simulink model "Modell_V5"  (R2014a)
settings: Solver=ode45  StartTime=0.0  StopTime=2  RelTol=1e-10
values from neighbouring files (symbols this model uses):
  AP = [pi 0 pi 0]'    [testscript.m]
  M_AP = 0    [testscript.m]
  stPendel = block.DialogPrm(1).Data    [systemPendel_V3.m]    (also in testscript.m = ladePendel())
  stTraj = berechneTrajektorie( stPendel, Q, R, T)    [testscript.m]
  x0 = block.DialogPrm(2).Data    [systemPendel_V3.m]    (also in testscript.m = [ 0 0 0 0]')
settings Model: Creator=asacakli  LastModifiedBy=Andreas
settings DataIOCC: SaveFormat=Dataset
settings OptimizationCC: SimCompilerOptimization=off
settings DebuggingCC: MergeDetectMultiDrivingBlocksExec=error  SolverPrmCheckMsg=none  FrameProcessingCompatibilityMsg=error  AllowSymbolicDim=off
settings HardwareCC: ProdBitPerPointer=64  ProdLargestAtomicFloat=Float  ProdIntDivRoundTo=Zero  ProdEndianess=LittleEndian  ProdWordSize=64  ProdHWDeviceType=Intel->x86-64 (Windows64)
settings RTWCC: RTWCompilerOptimization=off
settings GRTTargetCC: GeneratePreprocessorConditionals=Use local settings
settings ConfigComp: CovMetricSettings=dw  CovHtmlReporting=on  CovSaveCumulativeToWorkspaceVar=on  CovSaveSingleToWorkspaceVar=on  CovExternalEMLEnable=off

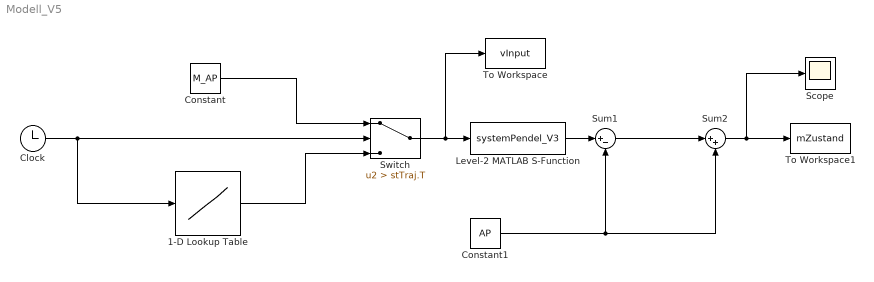
== system Modell_V5 ==
  1-D Lookup Table : Lookup_n-D  NumberOfTableDimensions=1  BreakpointsForDimension1=stTraj.vT  Table=stTraj.vU  InterpMethod=Cubic spline  ExtrapMethod=Clip  InternalRulePriority=Speed  RndMeth=Simplest  InputSameDT=on
  Clock : Clock
  Constant : Constant  Value=M_AP
  Constant1 : Constant  Value=AP
  Level-2 MATLAB S-Function : M-S-Function  FunctionName=systemPendel_V3  Parameters=stPendel,x0
  Scope : Scope
  Sum1 : Sum  Inputs=|+-
  Sum2 : Sum  Inputs=|++
  Switch : Switch  Criteria=u2 > Threshold  Threshold=stTraj.T
  To Workspace : ToWorkspace  VariableName=vInput  SaveFormat=Timeseries  SampleTime=-1
  To Workspace1 : ToWorkspace  VariableName=mZustand  SaveFormat=Timeseries  SampleTime=-1
  wires:
  Sum1/1 -> Sum2/1
  Constant1/1 -> Sum2/2, Sum1/2
  Level-2 MATLAB S-Function/1 -> Sum1/1
  Sum2/1 -> Scope/1, To Workspace1/1
  Switch/1 -> Level-2 MATLAB S-Function/1, To Workspace/1
  Clock/1 -> Switch/2, 1-D Lookup Table/1
  1-D Lookup Table/1 -> Switch/3
  Constant/1 -> Switch/1
